simulink subsystem "Subsystem_Odometria_ACT"  (R2023b)
settings: Solver=VariableStepAuto  StartTime=0.0  StopTime=10.0  RelTol=1e-3
undefined symbols (not defined in the file): DiscIntNeverNeededParam
settings Model: Creator=Alberto  LastModifiedBy=Alberto

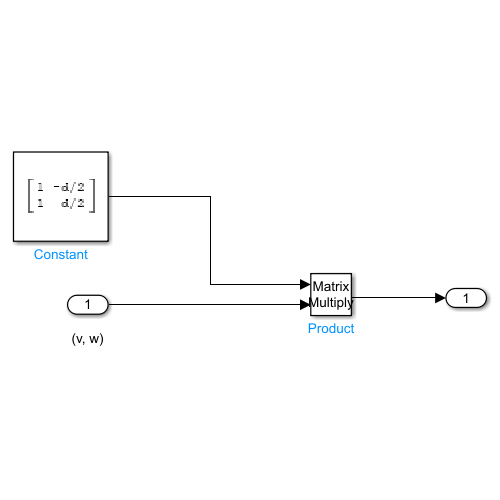
[thumbnail: Simulink's stored preview of the top-level diagram]
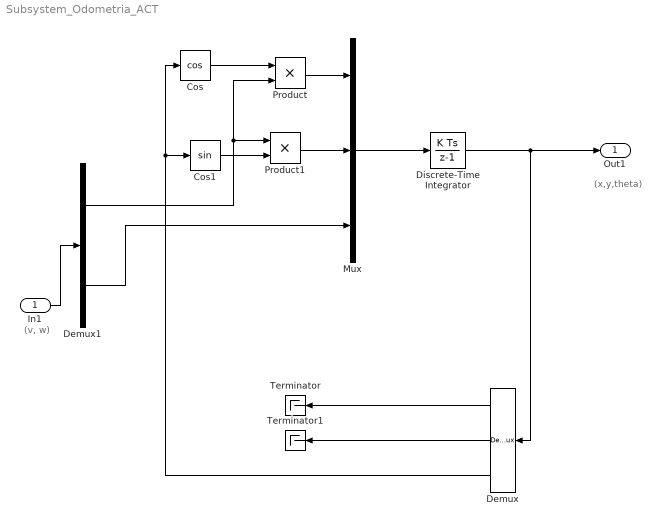
== system Subsystem_Odometria_ACT ==
  note: (x,y,theta)
  note: (v, w)
  In1 : Inport
  Cos : Trigonometry  Operator=cos
  Cos1 : Trigonometry
  Demux : Demux  Outputs=3
  Demux1 : Demux  Outputs=2
  Discrete-Time Integrator : DiscreteIntegrator  SampleTime=-1  ICPrevOutput=DiscIntNeverNeededParam  ICPrevScaledInput=DiscIntNeverNeededParam
  Mux : Mux  Inputs=3
  Product : Product
  Product1 : Product
  Terminator : Terminator
  Terminator1 : Terminator
  Out1 : Outport
  wires:
  Discrete-Time Integrator/1 -> Demux/1, Out1/1
  Demux/2 -> Terminator1/1
  Demux/1 -> Terminator/1
  In1/1 -> Demux1/1
  Demux/3 -> Cos1/1, Cos/1
  Cos/1 -> Product/1
  Cos1/1 -> Product1/2
  Demux1/1 -> Product1/1, Product/2
  Product/1 -> Mux/1
  Product1/1 -> Mux/2
  Demux1/2 -> Mux/3
  Mux/1 -> Discrete-Time Integrator/1
